simulink model "RT_TestMV"  (R2015b)
settings: Solver=FixedStepDiscrete  StartTime=0.0  StopTime=inf  FixedStep=samplePeriod  RelTol=1e-3
PreLoadFcn:
  | initialize;
  | scramInitialize;
  | KR_alpha;
  | Discrete_Compensator;
values from neighbouring files (symbols this model uses):
  a_sub = ones(DOF_sub,1)    [KR_alpha.m]
  A_sub = (dt*alpha1_sub)/(Msub-Msub*alpha3_sub)    [KR_alpha.m]
  a_sup = ones(DOF_sup,1)    [KR_alpha.m]
  A_sup = (dt*alpha1_sup)/(Msup-Msup*alpha3_sup)    [KR_alpha.m]
  a_vector = ones(DOF,1)    [KR_alpha.m]
  alpha_f_sub = rho_inf_sub/(rho_inf_sub+1)    (= 0.5)    [KR_alpha.m]
  alpha_f_sup = rho_inf_sup/(rho_inf_sup+1)    (= 0.5)    [KR_alpha.m]
  B_sub = ((1/dt)*Msub*alpha3_sub)/alpha1_sub    [KR_alpha.m]
  B_sup = ((1/dt)*Msup*alpha3_sup)/alpha1_sup    [KR_alpha.m]
  controlPeriod = 1/2048    (= 0.00048828125)    [initialize.m]
  Csub = betaKinit*Ksub    [KR_alpha.m]
  Csup = (2*0.01/w1)*Ksup    (= 0.00743030767319)    [KR_alpha.m]
  D_sub = inv(alpha1_sub)/dt    [KR_alpha.m]
  D_sup = inv(alpha1_sup)/dt    [KR_alpha.m]
  dt = samplePeriod    [KR_alpha.m]
  g = 386.089    [KR_alpha.m]
  gamma_sub = 0.5-alpha_m_sub+alpha_f_sub    (= 0.5)    [KR_alpha.m]
  gamma_sup = 0.5-alpha_m_sup+alpha_f_sup    (= 0.5)    [KR_alpha.m]
  K1 = 4.6686*K2    (= 9.3372)    [KR_alpha.m]
  K2 = 0.5*4    (= 2)    [KR_alpha.m]
  Ksub = Kstory    [KR_alpha.m]
  Msub = (0.88585/(56/450))*Mstory    (= 1.03248862309)    [KR_alpha.m]
  Msup = Mstory    (= 0.145044277356)    [KR_alpha.m]
  nAct = 4    [initialize.m]
  nDout = 4    [initialize.m]
  onesec = ceil(1/samplePeriod)    [Discrete_Compensator.m]
  samplePeriod = controlPeriod/upsampleFactor    (= 0.00048828125)    [initialize.m]
  scale_GM = 1.50    (= 1.5)    [KR_alpha.m]
  uy = 0.85    [KR_alpha.m]
undefined symbols (not defined in the file or in its folder): a, DiscIntNeverNeededParam, Gain_noise, lhpNode, stsNode
undefined symbols (not defined in the file): HybridCtrlParameters
libraries: simulink x16, slrtlib x12, xpcsystranlib x5
CloseFcn:
  | rtwprivate ssgencode ModelCloseRequest scrnet_receiver
settings Model: SimulationMode=external  ExtModeArmWhenConnect=off  Creator=mvetsch  LastModifiedBy=Analyst-UCSD
settings SolverCC: EnableConcurrentExecution=on
settings DataIOCC: LimitDataPoints=off  SaveFormat=Array  SignalLoggingSaveFormat=ModelDataLogs  SignalLoggingName=sigsOut
settings OptimizationCC: BlockReduction=off  BooleanDataType=off  OptimizeBlockIOStorage=off  BufferReuse=off  GlobalBufferReuse=off  ExpressionFolding=off  ExpressionDepthLimit=2147483647  LocalBlockOutputs=off  InitFltsAndDblsToZero=on
settings DebuggingCC: SaveWithParameterizedLinksMsg=none  UnderspecifiedInitializationDetection=Classic  MergeDetectMultiDrivingBlocksExec=none  SignalResolutionControl=TryResolveAllWithWarning  MultiTaskDSMMsg=warning  MultiTaskCondExecSysMsg=none  FcnCallInpInsideContextMsg=UseLocalSettings  StateNameClashWarn=warning
settings HardwareCC: ProdBitPerPointer=32  ProdLargestAtomicFloat=None  ProdWordSize=32  ProdLongLongMode=on  ProdHWDeviceType=Generic->32-bit x86 compatible
settings RTWCC: SystemTargetFile=slrt.tlc  TemplateMakefile=slrt_default_tmf  Description=Simulink Real-Time  RTWCompilerOptimization=on
settings SimulinkRealTimeCC: TargetFcnLib=ansi_tfl_tmw.mat  RL32LogBufSizeModifier=10000000  RL32IRQSourceModifier=Auto (PCI only)  xPCIRQSourceBoard=Scramnet_SC150+
settings ConfigComp: CovModelRefEnable=Off

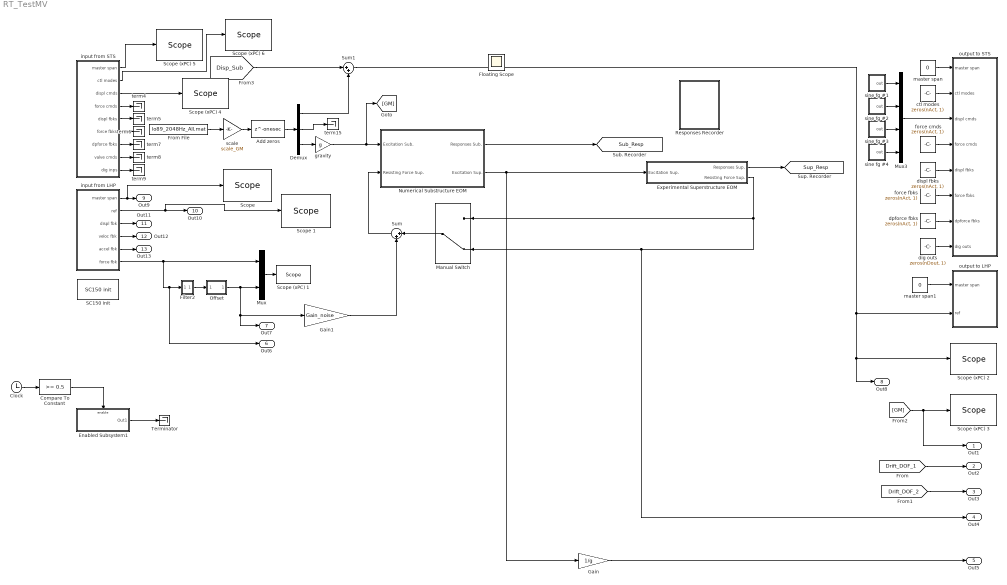
== system RT_TestMV ==
  Add zeros : Delay  DelayLength=onesec  InitialCondition=0
  Clock : Clock
  Compare To Constant : simulink/Logic and Bit Operations/Compare To Constant  relop=>=  const=0.5  OutDataTypeStr=boolean
  Demux : Demux  Outputs=3
  Enabled Subsystem1 : Subsystem  TreatAsAtomicUnit=on
  Experimental Superstructure EOM : Subsystem
  Filter2 : Subsystem
  From File : FromFile  FileName=lo89_2048Hz_All.mat  SampleTime=samplePeriod
  Gain : Gain  Gain=1/g
  Gain1 : Gain  Gain=Gain_noise
  Manual Switch : ManualSwitch  CurrentSetting=0
  Mux : Mux  Inputs=2
  Mux3 : Mux  Inputs=nAct
  Numerical Substructure EOM : Subsystem
  Offset : Subsystem  mask(Signal Offset){nS=HybridCtrlParameters.nDOF, nOffset=onesec}
      mask prompts: nS "Number of Signals: nS"; nOffset "Number of samples to initialize offset: nOffset"
      mask help:
      | Offset signal by average of signal over initial number of samples.
      | Set nOffset = -1 for no signal offset.
      mask Display: fprintf('Signal\nOffset')
  Responses Recorder : Subsystem
  SC150 init : xpcsystranlib/Shared Memory/SC150 init   node=node  pci=-1
  "Scope " : slrtlib/Displays and Logging/Scope   scopeno=8  scopetype=Target  autostart=on  viewmode=Numerical  formatstr='%15.6f'  grid=on  ylimits=[0,0]  nosamples=250  noprepostsamples=0  interleave=1  triggermode=FreeRun  triggersignal=1  trigsignalfromport=off  triggerlevel=0.0  triggerslope=Either  triggerscope=1  triggersample=0  filename=data.dat  mode=Lazy  writesize=512  autorestart=off  dynamicfilemode=off  maxwritefilesize=512*1024^2
  Scope (xPC) 1 : slrtlib/Displays and Logging/Scope   scopeno=2  scopetype=Target  autostart=on  viewmode=Graphical redraw  formatstr='%15.6f'  grid=on  ylimits=[0,0]  nosamples=1024  noprepostsamples=0  interleave=1  triggermode=FreeRun  triggersignal=1  trigsignalfromport=off  triggerlevel=0.0  triggerslope=Either  triggerscope=1  triggersample=0  filename=data.dat  mode=Lazy  writesize=512  autorestart=off  dynamicfilemode=off  maxwritefilesize=512*1024^2
  Scope (xPC) 2 : slrtlib/Displays and Logging/Scope   scopeno=3  scopetype=Target  autostart=on  viewmode=Graphical redraw  formatstr='%15.6f'  grid=on  ylimits=[0,0]  nosamples=1024  noprepostsamples=0  interleave=1  triggermode=FreeRun  triggersignal=1  trigsignalfromport=off  triggerlevel=0.0  triggerslope=Either  triggerscope=1  triggersample=0  filename=data.dat  mode=Lazy  writesize=512  autorestart=off  dynamicfilemode=off  maxwritefilesize=512*1024^2
  Scope (xPC) 3 : slrtlib/Displays and Logging/Scope   scopeno=4  scopetype=Target  autostart=on  viewmode=Graphical redraw  formatstr='%15.6f'  grid=on  ylimits=[0,0]  nosamples=1024  noprepostsamples=0  interleave=1  triggermode=FreeRun  triggersignal=1  trigsignalfromport=off  triggerlevel=0.0  triggerslope=Either  triggerscope=1  triggersample=0  filename=data.dat  mode=Lazy  writesize=512  autorestart=off  dynamicfilemode=off  maxwritefilesize=512*1024^2
  Scope (xPC) 4 : slrtlib/Displays and Logging/Scope   scopeno=1  scopetype=Target  autostart=on  viewmode=Numerical  formatstr='%15.6f'  grid=on  ylimits=[0,0]  nosamples=1024  noprepostsamples=0  interleave=1  triggermode=FreeRun  triggersignal=1  trigsignalfromport=off  triggerlevel=0.0  triggerslope=Either  triggerscope=1  triggersample=0  filename=data.dat  mode=Lazy  writesize=512  autorestart=off  dynamicfilemode=off  maxwritefilesize=512*1024^2
  Scope (xPC) 5 : slrtlib/Displays and Logging/Scope   scopeno=5  scopetype=Target  autostart=on  viewmode=Numerical  formatstr='%15.6f'  grid=on  ylimits=[0,0]  nosamples=1024  noprepostsamples=0  interleave=1  triggermode=FreeRun  triggersignal=1  trigsignalfromport=off  triggerlevel=0.0  triggerslope=Either  triggerscope=1  triggersample=0  filename=data.dat  mode=Lazy  writesize=512  autorestart=off  dynamicfilemode=off  maxwritefilesize=512*1024^2
  Scope (xPC) 6 : slrtlib/Displays and Logging/Scope   scopeno=6  scopetype=Target  autostart=on  viewmode=Numerical  formatstr='%15.6f'  grid=on  ylimits=[0,0]  nosamples=1024  noprepostsamples=0  interleave=1  triggermode=FreeRun  triggersignal=1  trigsignalfromport=off  triggerlevel=0.0  triggerslope=Either  triggerscope=1  triggersample=0  filename=data.dat  mode=Lazy  writesize=512  autorestart=off  dynamicfilemode=off  maxwritefilesize=512*1024^2
  Scope 1 : slrtlib/Displays and Logging/Scope   scopeno=7  scopetype=Target  autostart=on  viewmode=Graphical redraw  formatstr='%15.6f'  grid=on  ylimits=[0,0]  nosamples=250  noprepostsamples=0  interleave=1  triggermode=FreeRun  triggersignal=1  trigsignalfromport=off  triggerlevel=0.0  triggerslope=Either  triggerscope=1  triggersample=0  filename=data.dat  mode=Lazy  writesize=512  autorestart=off  dynamicfilemode=off  maxwritefilesize=512*1024^2
  Sum : Sum  Inputs=|++
  Sum1 : Sum  Inputs=|++
  Terminator : Terminator
  ctl modes : Constant  Value=zeros(nAct, 1)
  dig outs : Constant  Value=zeros(nDout, 1)  OutDataTypeStr=uint32
  displ fbks : Constant  Value=zeros(nAct, 1)
  dpforce fbks : Constant  Value=zeros(nAct, 1)
  force cmds : Constant  Value=zeros(nAct, 1)
  force fbks : Constant  Value=zeros(nAct, 1)
  gravity : Gain  Gain=g
  input from LHP : Subsystem
  input from STS : Subsystem
  master span : Constant  Value=0
  master span1 : Constant  Value=0
  output to LHP : Subsystem
  output to STS : Subsystem
  scale : Gain  Gain=scale_GM
  sine fg #1 : Subsystem  mask(Sine Function Generator){ampl=0.5, freq=1, spanInterval=1, samplePeriod=controlPeriod}
      mask prompts: ampl "Amplitude"; freq "Frequency (Hz)"; spanInterval "Span interval (sec)"; samplePeriod "Sample period (sec)"
  sine fg #2 : Subsystem  mask(Sine Function Generator){ampl=0.5, freq=2, spanInterval=1, samplePeriod=controlPeriod}
      mask prompts: ampl "Amplitude"; freq "Frequency (Hz)"; spanInterval "Span interval (sec)"; samplePeriod "Sample period (sec)"
  sine fg #3 : Subsystem  mask(Sine Function Generator){ampl=0.5, freq=3, spanInterval=1, samplePeriod=controlPeriod}
      mask prompts: ampl "Amplitude"; freq "Frequency (Hz)"; spanInterval "Span interval (sec)"; samplePeriod "Sample period (sec)"
  sine fg #4 : Subsystem  mask(Sine Function Generator){ampl=0.5, freq=4, spanInterval=1, samplePeriod=controlPeriod}
      mask prompts: ampl "Amplitude"; freq "Frequency (Hz)"; spanInterval "Span interval (sec)"; samplePeriod "Sample period (sec)"
  term{4..9,15} (7 alike) : Terminator
  Out1 : Outport  SampleTime=samplePeriod
  Out2 : Outport  Port=2  SampleTime=samplePeriod
  Out3 : Outport  Port=3  SampleTime=samplePeriod
  Out4 : Outport  Port=4  SampleTime=samplePeriod
  Out5 : Outport  Port=5  SampleTime=samplePeriod
  Out6 : Outport  Port=6  SampleTime=samplePeriod
  Out7 : Outport  Port=7  SampleTime=samplePeriod
  Out8 : Outport  Port=8  SampleTime=samplePeriod
  Out9 : Outport  Port=9  SampleTime=samplePeriod
  Out10 : Outport  Port=10  SampleTime=samplePeriod
  Out11 : Outport  Port=11  SampleTime=samplePeriod
  Out12 : Outport  Port=12  SampleTime=samplePeriod
  Out13 : Outport  Port=13  SampleTime=samplePeriod
  Floating Scope : Scope
  tag scope: Sub_Resp=global, Sup_Resp=global
  wires:
  master span/1 -> output to STS/1(master span)
  ctl modes/1 -> output to STS/2(ctl modes)
  force cmds/1 -> output to STS/4(force cmds)
  sine fg #1/1(out) -> Mux3/1
  sine fg #2/1(out) -> Mux3/2
  displ fbks/1 -> output to STS/5(displ fbks)
  force fbks/1 -> output to STS/6(force fbks)
  dpforce fbks/1 -> output to STS/7(dpforce fbks)
  input from STS/2(ctl modes) -> Scope (xPC) 6/1
  input from STS/4(force cmds) -> term4/1
  input from STS/5(displ fbks) -> term5/1
  input from STS/6(force fbks) -> term6/1
  input from STS/7(dpforce fbks) -> term7/1
  input from STS/8(valve cmds) -> term8/1
  input from STS/9(dig inps) -> term9/1
  dig outs/1 -> output to STS/8(dig outs)
  Mux3/1 -> output to STS/3(displ cmds)
  sine fg #3/1(out) -> Mux3/3
  sine fg #4/1(out) -> Mux3/4
  input from LHP/1(master span) -> "Scope "/1, Out9/1
  input from LHP/3(displ fbk) -> Out11/1
  input from LHP/4(veloc fbk) -> Out12/1
  input from LHP/5(accel fbk) -> Out13/1
  Mux/1 -> Scope (xPC) 1/1
  input from LHP/6(force fbk) -> Out6/1, Filter2/1(In1), Mux/1
  Numerical Substructure EOM/1(Responses Sub.) -> [Sub_Resp]
  Experimental Superstructure EOM/1(Responses Sup.) -> [Sup_Resp]
  [Drift_DOF_1] -> Out2/1
  [Drift_DOF_2] -> Out3/1
  master span1/1 -> output to LHP/1(master span)
  Filter2/1(Out1) -> Offset/1(In1)
  Offset/1(Out1) -> Out7/1, Gain1/1, Mux/2
  input from LHP/2(ref) -> Scope 1/1, Out10/1
  Experimental Superstructure EOM/2(Resisting Force Sup.) -> Manual Switch/1, Manual Switch/2, Out4/1
  From File/1 -> scale/1
  gravity/1 -> [GM], Numerical Substructure EOM/1(Excitation Sub.)
  Sum/1 -> Numerical Substructure EOM/2(Resisting Force Sup.)
  Manual Switch/1 -> Sum/1
  [GM] -> Out1/1, Scope (xPC) 3/1
  Numerical Substructure EOM/2(Excitation Sup.) -> Experimental Superstructure EOM/1(Excitation Sup.), Gain/1
  Gain1/1 -> Sum/2
  Add zeros/1 -> Demux/1
  Demux/3 -> gravity/1
  Demux/2 -> term15/1
  [Disp_Sub] -> Sum1/1
  Demux/1 -> Sum1/2
  Gain/1 -> Out5/1
  scale/1 -> Add zeros/1
  input from STS/1(master span) -> Scope (xPC) 5/1
  input from STS/3(displ cmds) -> Scope (xPC) 4/1
  Sum1/1 -> Out8/1, Scope (xPC) 2/1, output to LHP/2(ref)
  Compare To Constant/1 -> Enabled Subsystem1/Enable
  Clock/1 -> Compare To Constant/1
  Enabled Subsystem1/1(Out1) -> Terminator/1

== system RT_TestMV/Enabled Subsystem1 ==
  Enable : EnablePort
  sine fg #5 : Subsystem  mask(Sine Function Generator){ampl=1, freq=1, spanInterval=1, samplePeriod=-1}
      mask prompts: ampl "Amplitude"; freq "Frequency (Hz)"; spanInterval "Span interval (sec)"; samplePeriod "Sample period (sec)"
  Out1 : Outport
  wires:
  sine fg #5/1(out) -> Out1/1

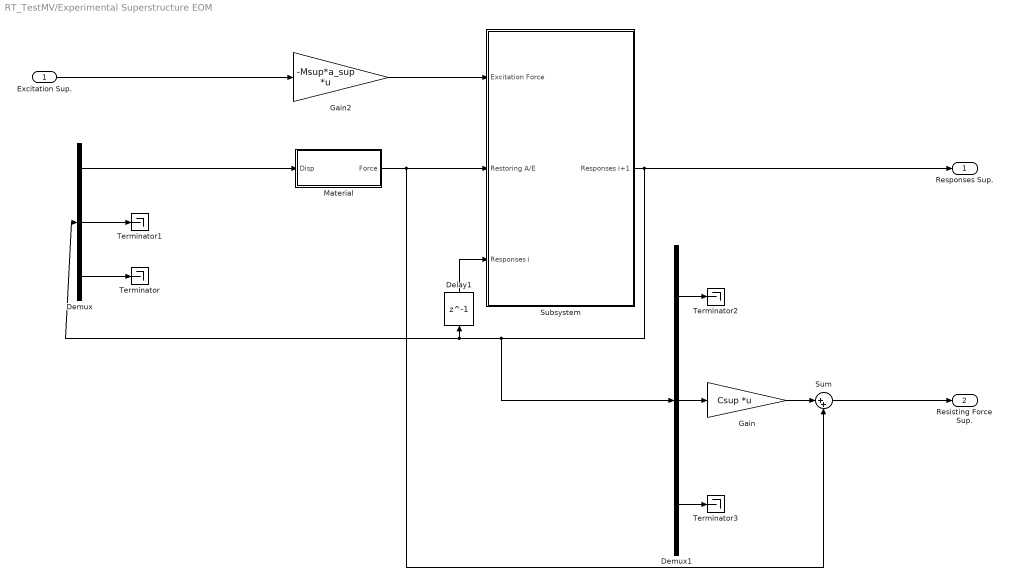
== system RT_TestMV/Experimental Superstructure EOM ==
  Excitation Sup. : Inport
  Delay1 : Delay  DelayLength=1
  Demux : Demux  Outputs=3
  Demux1 : Demux  Outputs=3
  Gain : Gain  Gain=Csup  Multiplication=Matrix(K*u) (u vector)
  Gain2 : Gain  Gain=-Msup*a_sup  Multiplication=Matrix(K*u)
  Material : Subsystem
  Subsystem : Subsystem
  Sum : Sum  Inputs=|++
  Terminator{,1..3} (4 alike) : Terminator
  Responses Sup. : Outport
  Resisting Force Sup. : Outport  Port=2
  wires:
  Subsystem/1(Responses i+1) -> Demux1/1, Demux/1, Delay1/1, Responses Sup./1
  Excitation Sup./1 -> Gain2/1
  Demux1/2 -> Gain/1
  Sum/1 -> Resisting Force Sup./1
  Demux/1 -> Material/1(Disp)
  Demux/3 -> Terminator/1
  Demux/2 -> Terminator1/1
  Demux1/1 -> Terminator2/1
  Demux1/3 -> Terminator3/1
  Gain/1 -> Sum/1
  Delay1/1 -> Subsystem/3(Responses i)
  Material/1(Force) -> Sum/2, Subsystem/2(Restoring A/E)
  Gain2/1 -> Subsystem/1(Excitation Force)

== system RT_TestMV/Filter2 ==
  In1 : Inport
  MovingAverage Filter2 : DiscreteFir  Coefficients=1/numSample*ones(1,numSample)  mask(Moving Average Filter){numSample=7}
      mask prompts: numSample "Number of Samples: numSample"
      mask help:
      | Moving average filter by using discrete FIR filter.
      | Set numSample = 1 for no filtering.
      mask Display: fprintf('MovingAverage\nFilter')
  Out1 : Outport
  wires:
  In1/1 -> MovingAverage Filter2/1
  MovingAverage Filter2/1 -> Out1/1

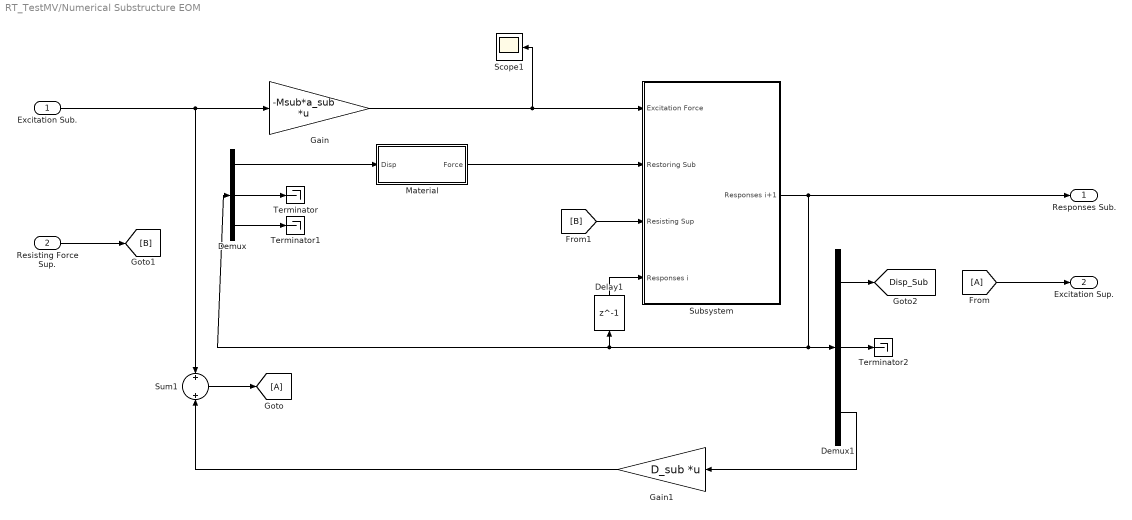
== system RT_TestMV/Numerical Substructure EOM ==
  Excitation Sub. : Inport
  Resisting Force Sup. : Inport  Port=2
  Delay1 : Delay  DelayLength=1
  Demux : Demux  Outputs=3
  Demux1 : Demux  Outputs=3
  Gain : Gain  Gain=-Msub*a_sub  Multiplication=Matrix(K*u)
  Gain1 : Gain  Gain=D_sub  Multiplication=Matrix(K*u) (u vector)
  Material : Subsystem
  Scope1 : Scope
  Subsystem : Subsystem
  Sum1 : Sum  Inputs=+||+
  Terminator : Terminator
  Terminator1 : Terminator
  Terminator2 : Terminator
  Responses Sub. : Outport
  Excitation Sup. : Outport  Port=2
  tag scope: Disp_Sub=global
  wires:
  Gain/1 -> Scope1/1, Subsystem/1(Excitation Force)
  Subsystem/1(Responses i+1) -> Demux/1, Delay1/1, Demux1/1, Responses Sub./1
  Demux/1 -> Material/1(Disp)
  Excitation Sub./1 -> Sum1/1, Gain/1
  Demux1/3 -> Gain1/1
  Demux/2 -> Terminator/1
  Demux/3 -> Terminator1/1
  Demux1/1 -> [Disp_Sub]
  Delay1/1 -> Subsystem/4(Responses i)
  Material/1(Force) -> Subsystem/2(Restoring Sub)
  Gain1/1 -> Sum1/2
  Demux1/2 -> Terminator2/1
  Sum1/1 -> [A]
  [A] -> Excitation Sup./1
  Resisting Force Sup./1 -> [B]
  [B] -> Subsystem/3(Resisting Sup)

== system RT_TestMV/Offset ==
  In1 : Inport
  Constant : Constant  Value=zeros(1,nS)
  Counter : simulink/Sources/Counter Free-Running  NumBits=32  tsamp=-1
  Data Store Memory : DataStoreMemory  DataStoreName=x0  InitialValue=zeros(1,nS)  OutDataTypeStr=double
  Data Store Read : DataStoreRead  DataStoreName=x0  SampleTime=controlPeriod
  If : If  IfExpression=u1 < nOffset  ShowElse=off
  If Action : Subsystem  TreatAsAtomicUnit=on
  Sum1 : Sum  Inputs=+-|  SaturateOnIntegerOverflow=on  InputSameDT=on  OutDataTypeStr=Inherit: Same as first input
  Switch : Switch  Threshold=nOffset  SaturateOnIntegerOverflow=on  InputSameDT=on
  typeConv2 : DataTypeConversion  OutDataTypeStr=double  SaturateOnIntegerOverflow=on  RndMeth=Zero
  Out1 : Outport
  wires:
  Switch/1 -> Out1/1
  Sum1/1 -> Switch/1
  Data Store Read/1 -> Sum1/2
  In1/1 -> If Action/1(In1), Sum1/1
  Constant/1 -> Switch/3
  Counter/1 -> typeConv2/1
  If/1 -> If Action/Action
  typeConv2/1 -> Switch/2, If/1

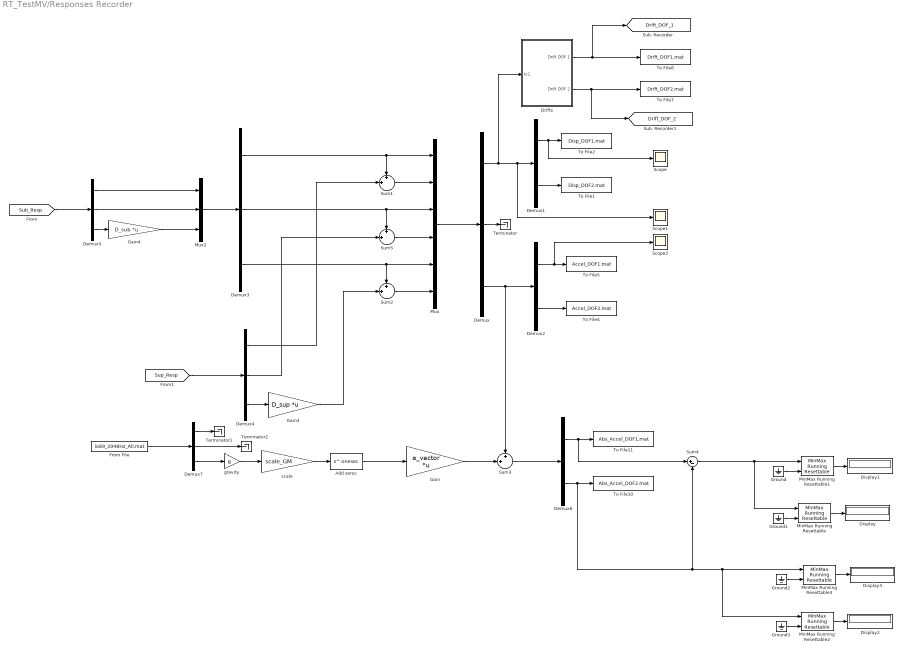
== system RT_TestMV/Responses Recorder ==
  Add zeros : Delay  DelayLength=onesec  InitialCondition=0
  Demux{,3..5,7} (5 alike) : Demux  Outputs=3
  Demux1 : Demux  Outputs=2
  Demux2 : Demux  Outputs=2
  Demux6 : Demux  Outputs=2
  Display{,1..3} (4 alike) : Display
  Drifts : Subsystem
  From File : FromFile  FileName=lo89_2048Hz_All.mat  SampleTime=samplePeriod
  Gain : Gain  Gain=a_vector  Multiplication=Matrix(K*u)
  Gain3 : Gain  Gain=D_sup  Multiplication=Matrix(K*u) (u vector)
  Gain4 : Gain  Gain=D_sub  Multiplication=Matrix(K*u) (u vector)
  Ground{,1..3} (4 alike) : Ground
  MinMax Running Resettable : simulink/Math Operations/MinMax Running Resettable  Function=max  vinit=0.0
  MinMax Running Resettable1 : simulink/Math Operations/MinMax Running Resettable  Function=min  vinit=0.0
  MinMax Running Resettable2 : simulink/Math Operations/MinMax Running Resettable  Function=max  vinit=0.0
  MinMax Running Resettable3 : simulink/Math Operations/MinMax Running Resettable  Function=min  vinit=0.0
  Mux : Mux  Inputs=6
  Mux2 : Mux  Inputs=3
  Scope : Scope
  Scope1 : Scope
  Scope2 : Scope
  Sum{1..3,5} (4 alike) : Sum  Inputs=+|+||
  Sum4 : Sum  Inputs=|+-
  Terminator : Terminator
  Terminator1 : Terminator
  Terminator2 : Terminator
  To File1 : ToFile  Filename=Disp_DOF2.mat
  To File10 : ToFile  Filename=Abs_Accel_DOF2.mat
  To File11 : ToFile  Filename=Abs_Accel_DOF1.mat
  To File2 : ToFile  Filename=Disp_DOF1.mat
  To File4 : ToFile  Filename=Accel_DOF2.mat
  To File5 : ToFile  Filename=Accel_DOF1.mat
  To File7 : ToFile  Filename=Drift_DOF2.mat  MatrixName=Drift_DOF2
  To File8 : ToFile  Filename=Drift_DOF1.mat  MatrixName=Drift_DOF1
  gravity : Gain  Gain=g
  scale : Gain  Gain=scale_GM
  tag scope: Drift_DOF_1=global, Drift_DOF_2=global
  wires:
  Demux1/2 -> To File1/1
  Demux2/1 -> Scope2/1, To File5/1
  Demux/3 -> Sum3/1, Demux2/1
  Demux1/1 -> Scope/1, To File2/1
  Demux/1 -> Drifts/1(In1), Scope1/1, Demux1/1
  [Sup_Resp] -> Demux4/1
  Mux/1 -> Demux/1
  Demux3/3 -> Sum2/1, Mux/5
  Demux4/3 -> Gain3/1
  Sum2/1 -> Mux/6
  Gain3/1 -> Sum2/2
  [Sub_Resp] -> Demux5/1
  Demux5/2 -> Mux2/2
  Demux5/1 -> Mux2/1
  Demux5/3 -> Gain4/1
  Gain4/1 -> Mux2/3
  Mux2/1 -> Demux3/1
  Demux/2 -> Terminator/1
  MinMax Running Resettable/1 -> Display/1
  MinMax Running Resettable1/1 -> Display1/1
  Ground/1 -> MinMax Running Resettable1/2
  Ground1/1 -> MinMax Running Resettable/2
  Demux2/2 -> To File4/1
  MinMax Running Resettable2/1 -> Display2/1
  MinMax Running Resettable3/1 -> Display3/1
  Ground2/1 -> MinMax Running Resettable3/2
  Ground3/1 -> MinMax Running Resettable2/2
  Drifts/1(Drift DOF 1) -> [Drift_DOF_1], To File8/1
  Drifts/2(Drift DOF 2) -> [Drift_DOF_2], To File7/1
  gravity/1 -> scale/1
  Gain/1 -> Sum3/2
  Sum3/1 -> Demux6/1
  scale/1 -> Add zeros/1
  Demux3/1 -> Sum1/1, Mux/1
  Demux4/1 -> Sum1/2
  Sum1/1 -> Mux/2
  Demux3/2 -> Sum5/1, Mux/3
  Demux4/2 -> Sum5/2
  Sum5/1 -> Mux/4
  Demux6/1 -> Sum4/1, To File11/1
  Demux6/2 -> Sum4/2, MinMax Running Resettable2/1, MinMax Running Resettable3/1, To File10/1
  Sum4/1 -> MinMax Running Resettable/1, MinMax Running Resettable1/1
  Add zeros/1 -> Gain/1
  Demux7/3 -> gravity/1
  From File/1 -> Demux7/1
  Demux7/1 -> Terminator1/1
  Demux7/2 -> Terminator2/1

== system RT_TestMV/input from LHP ==
  SC150 read : xpcsystranlib/Shared Memory/SC150 read   partition=lhpNode.Partitions(3:end)  errorport=off  ts=controlPeriod  pci=-1
  SC150 unpack : slrtlib/Shared Memory/Shared Memory Unpack   partition=lhpNode.Partitions(3:end)
  typeConv{1..6} (6 alike) : DataTypeConversion  OutDataTypeStr=double  SaturateOnIntegerOverflow=on  RndMeth=Zero
  master span : Outport
  ref : Outport  Port=2
  displ fbk : Outport  Port=3
  veloc fbk : Outport  Port=4
  accel fbk : Outport  Port=5
  force fbk : Outport  Port=6
  wires:
  SC150 unpack/6 -> typeConv6/1
  SC150 unpack/5 -> typeConv5/1
  SC150 unpack/4 -> typeConv4/1
  SC150 unpack/3 -> typeConv3/1
  SC150 unpack/2 -> typeConv2/1
  typeConv6/1 -> force fbk/1
  typeConv5/1 -> accel fbk/1
  typeConv4/1 -> veloc fbk/1
  typeConv3/1 -> displ fbk/1
  typeConv1/1 -> master span/1
  SC150 read/1 -> SC150 unpack/1
  typeConv2/1 -> ref/1
  SC150 unpack/1 -> typeConv1/1

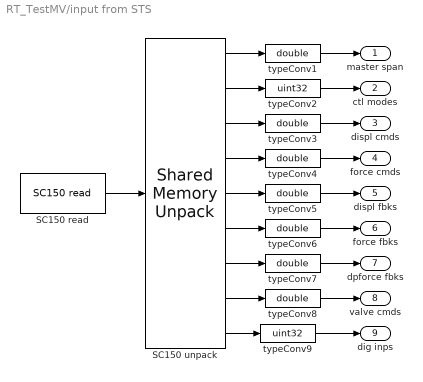
== system RT_TestMV/input from STS ==
  SC150 read : xpcsystranlib/Shared Memory/SC150 read   partition=stsNode.Partitions(9:end)  errorport=off  ts=controlPeriod  pci=-1
  SC150 unpack : slrtlib/Shared Memory/Shared Memory Unpack   partition=stsNode.Partitions(9:end)
  typeConv{1,3..8} (7 alike) : DataTypeConversion  OutDataTypeStr=double  SaturateOnIntegerOverflow=on  RndMeth=Zero
  typeConv2 : DataTypeConversion  OutDataTypeStr=uint32  SaturateOnIntegerOverflow=on  RndMeth=Zero
  typeConv9 : DataTypeConversion  OutDataTypeStr=uint32  SaturateOnIntegerOverflow=on  RndMeth=Zero
  master span : Outport
  ctl modes : Outport  Port=2
  displ cmds : Outport  Port=3
  force cmds : Outport  Port=4
  displ fbks : Outport  Port=5
  force fbks : Outport  Port=6
  dpforce fbks : Outport  Port=7
  valve cmds : Outport  Port=8
  dig inps : Outport  Port=9
  wires:
  SC150 unpack/8 -> typeConv8/1
  SC150 unpack/7 -> typeConv7/1
  SC150 unpack/6 -> typeConv6/1
  SC150 unpack/5 -> typeConv5/1
  SC150 unpack/4 -> typeConv4/1
  SC150 unpack/2 -> typeConv2/1
  typeConv2/1 -> ctl modes/1
  SC150 read/1 -> SC150 unpack/1
  typeConv1/1 -> master span/1
  typeConv3/1 -> displ cmds/1
  typeConv4/1 -> force cmds/1
  typeConv5/1 -> displ fbks/1
  typeConv6/1 -> force fbks/1
  typeConv7/1 -> dpforce fbks/1
  typeConv8/1 -> valve cmds/1
  SC150 unpack/9 -> typeConv9/1
  typeConv9/1 -> dig inps/1
  SC150 unpack/3 -> typeConv3/1
  SC150 unpack/1 -> typeConv1/1

== system RT_TestMV/output to LHP ==
  master span : Inport
  ref : Inport  Port=2
  SC150 pack : slrtlib/Shared Memory/Shared Memory Pack   partition=lhpNode.Partitions(1:2)
  SC150 write : xpcsystranlib/Shared Memory/SC150 write   partition=lhpNode.Partitions(1:2)  errorport=off  ts=controlPeriod  pci=-1
  typeConv1 : DataTypeConversion  OutDataTypeStr=single  SaturateOnIntegerOverflow=on  RndMeth=Zero
  typeConv2 : DataTypeConversion  OutDataTypeStr=single  SaturateOnIntegerOverflow=on  RndMeth=Zero
  wires:
  master span/1 -> typeConv1/1
  SC150 pack/1 -> SC150 write/1
  ref/1 -> typeConv2/1
  typeConv1/1 -> SC150 pack/1
  typeConv2/1 -> SC150 pack/2

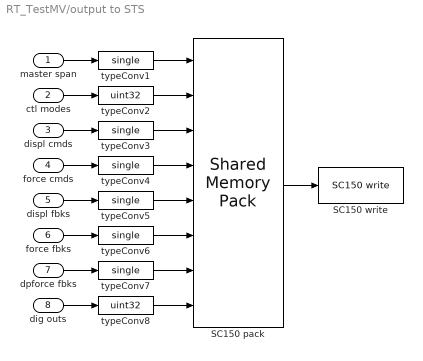
== system RT_TestMV/output to STS ==
  master span : Inport
  ctl modes : Inport  Port=2
  displ cmds : Inport  Port=3
  force cmds : Inport  Port=4
  displ fbks : Inport  Port=5
  force fbks : Inport  Port=6
  dpforce fbks : Inport  Port=7
  dig outs : Inport  Port=8
  SC150 pack : slrtlib/Shared Memory/Shared Memory Pack   partition=stsNode.Partitions(1:8)
  SC150 write : xpcsystranlib/Shared Memory/SC150 write   partition=stsNode.Partitions(1:8)  errorport=off  ts=controlPeriod  pci=-1
  typeConv{1,3..7} (6 alike) : DataTypeConversion  OutDataTypeStr=single  SaturateOnIntegerOverflow=on  RndMeth=Zero
  typeConv2 : DataTypeConversion  OutDataTypeStr=uint32  SaturateOnIntegerOverflow=on  RndMeth=Zero
  typeConv8 : DataTypeConversion  OutDataTypeStr=uint32  SaturateOnIntegerOverflow=on  RndMeth=Zero
  wires:
  typeConv4/1 -> SC150 pack/4
  typeConv3/1 -> SC150 pack/3
  typeConv2/1 -> SC150 pack/2
  typeConv1/1 -> SC150 pack/1
  ctl modes/1 -> typeConv2/1
  displ cmds/1 -> typeConv3/1
  SC150 pack/1 -> SC150 write/1
  master span/1 -> typeConv1/1
  force cmds/1 -> typeConv4/1
  displ fbks/1 -> typeConv5/1
  force fbks/1 -> typeConv6/1
  dpforce fbks/1 -> typeConv7/1
  typeConv5/1 -> SC150 pack/5
  typeConv6/1 -> SC150 pack/6
  typeConv7/1 -> SC150 pack/7
  typeConv8/1 -> SC150 pack/8
  dig outs/1 -> typeConv8/1

== system RT_TestMV/sine fg #1 ==
  Product : Product  SaturateOnIntegerOverflow=on  InputSameDT=on  OutDataTypeStr=Inherit: Same as first input
  integrator : DiscreteIntegrator  SampleTime=-1  LimitOutput=on  UpperSaturationLimit=1  LowerSaturationLimit=0  ICPrevOutput=DiscIntNeverNeededParam  ICPrevScaledInput=DiscIntNeverNeededParam
  sine : Sin  Amplitude=ampl  Frequency=2 * pi * freq  SampleTime=samplePeriod
  span rate : Constant  Value=1/spanInterval
  out : Outport
  wires:
  Product/1 -> out/1
  sine/1 -> Product/1
  span rate/1 -> integrator/1
  integrator/1 -> Product/2

== system RT_TestMV/sine fg #2 ==
  Product : Product  SaturateOnIntegerOverflow=on  InputSameDT=on  OutDataTypeStr=Inherit: Same as first input
  integrator : DiscreteIntegrator  SampleTime=-1  LimitOutput=on  UpperSaturationLimit=1  LowerSaturationLimit=0  ICPrevOutput=DiscIntNeverNeededParam  ICPrevScaledInput=DiscIntNeverNeededParam
  sine : Sin  Amplitude=ampl  Frequency=2 * pi * freq  SampleTime=samplePeriod
  span rate : Constant  Value=1/spanInterval
  out : Outport
  wires:
  integrator/1 -> Product/2
  span rate/1 -> integrator/1
  sine/1 -> Product/1
  Product/1 -> out/1

== system RT_TestMV/sine fg #3 ==
  Product : Product  SaturateOnIntegerOverflow=on  InputSameDT=on  OutDataTypeStr=Inherit: Same as first input
  integrator : DiscreteIntegrator  SampleTime=-1  LimitOutput=on  UpperSaturationLimit=1  LowerSaturationLimit=0  ICPrevOutput=DiscIntNeverNeededParam  ICPrevScaledInput=DiscIntNeverNeededParam
  sine : Sin  Amplitude=ampl  Frequency=2 * pi * freq  SampleTime=samplePeriod
  span rate : Constant  Value=1/spanInterval
  out : Outport
  wires:
  Product/1 -> out/1
  sine/1 -> Product/1
  span rate/1 -> integrator/1
  integrator/1 -> Product/2

== system RT_TestMV/sine fg #4 ==
  Product : Product  SaturateOnIntegerOverflow=on  InputSameDT=on  OutDataTypeStr=Inherit: Same as first input
  integrator : DiscreteIntegrator  SampleTime=-1  LimitOutput=on  UpperSaturationLimit=1  LowerSaturationLimit=0  ICPrevOutput=DiscIntNeverNeededParam  ICPrevScaledInput=DiscIntNeverNeededParam
  sine : Sin  Amplitude=ampl  Frequency=2 * pi * freq  SampleTime=samplePeriod
  span rate : Constant  Value=1/spanInterval
  out : Outport
  wires:
  integrator/1 -> Product/2
  span rate/1 -> integrator/1
  sine/1 -> Product/1
  Product/1 -> out/1

== system RT_TestMV/Enabled Subsystem1/sine fg #5 ==
  Product : Product  SaturateOnIntegerOverflow=on  InputSameDT=on  OutDataTypeStr=Inherit: Same as first input
  integrator : DiscreteIntegrator  SampleTime=-1  LimitOutput=on  UpperSaturationLimit=1  LowerSaturationLimit=0  ICPrevOutput=DiscIntNeverNeededParam  ICPrevScaledInput=DiscIntNeverNeededParam
  sine : Sin  Amplitude=ampl  Frequency=2 * pi * freq  SampleTime=samplePeriod
  span rate : Constant  Value=1/spanInterval
  out : Outport
  wires:
  integrator/1 -> Product/2
  span rate/1 -> integrator/1
  sine/1 -> Product/1
  Product/1 -> out/1

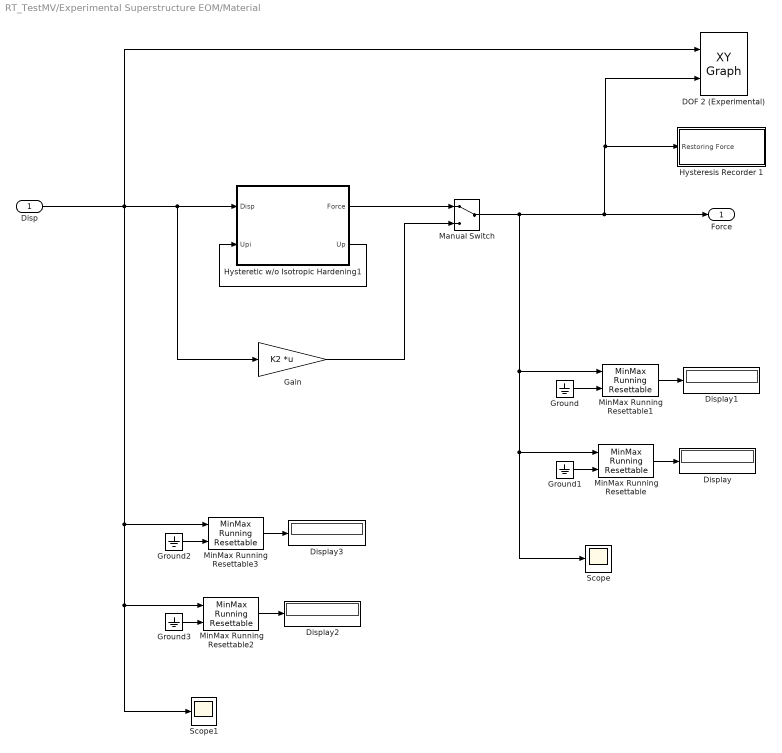
== system RT_TestMV/Experimental Superstructure EOM/Material ==
  Disp : Inport
  DOF 2 (Experimental) : simulink/Sinks/XY Graph  xmin=-6  xmax=6  ymin=-25  ymax=25  st=-1
  Display{,1..3} (4 alike) : Display
  Gain : Gain  Gain=K2  Multiplication=Matrix(K*u) (u vector)
  Ground{,1..3} (4 alike) : Ground
  Hysteresis Recorder 1 : Subsystem
  Hysteretic w/o Isotropic Hardening1 : Subsystem
  Manual Switch : ManualSwitch
  MinMax Running Resettable : simulink/Math Operations/MinMax Running Resettable  Function=max  vinit=0.0
  MinMax Running Resettable1 : simulink/Math Operations/MinMax Running Resettable  Function=min  vinit=0.0
  MinMax Running Resettable2 : simulink/Math Operations/MinMax Running Resettable  Function=max  vinit=0.0
  MinMax Running Resettable3 : simulink/Math Operations/MinMax Running Resettable  Function=min  vinit=0.0
  Scope : Scope
  Scope1 : Scope
  Force : Outport
  wires:
  Hysteretic w/o Isotropic Hardening1/2(Up) -> Hysteretic w/o Isotropic Hardening1/2(Upi)
  Hysteretic w/o Isotropic Hardening1/1(Force) -> Manual Switch/1
  Gain/1 -> Manual Switch/2
  MinMax Running Resettable2/1 -> Display2/1
  Ground/1 -> MinMax Running Resettable1/2
  Ground2/1 -> MinMax Running Resettable3/2
  Ground1/1 -> MinMax Running Resettable/2
  MinMax Running Resettable1/1 -> Display1/1
  MinMax Running Resettable/1 -> Display/1
  Ground3/1 -> MinMax Running Resettable2/2
  Manual Switch/1 -> MinMax Running Resettable1/1, MinMax Running Resettable/1, Scope/1, DOF 2 (Experimental)/2, Hysteresis Recorder 1/1(Restoring Force), Force/1
  MinMax Running Resettable3/1 -> Display3/1
  Disp/1 -> DOF 2 (Experimental)/1, MinMax Running Resettable3/1, MinMax Running Resettable2/1, Scope1/1, Gain/1, Hysteretic w/o Isotropic Hardening1/1(Disp)

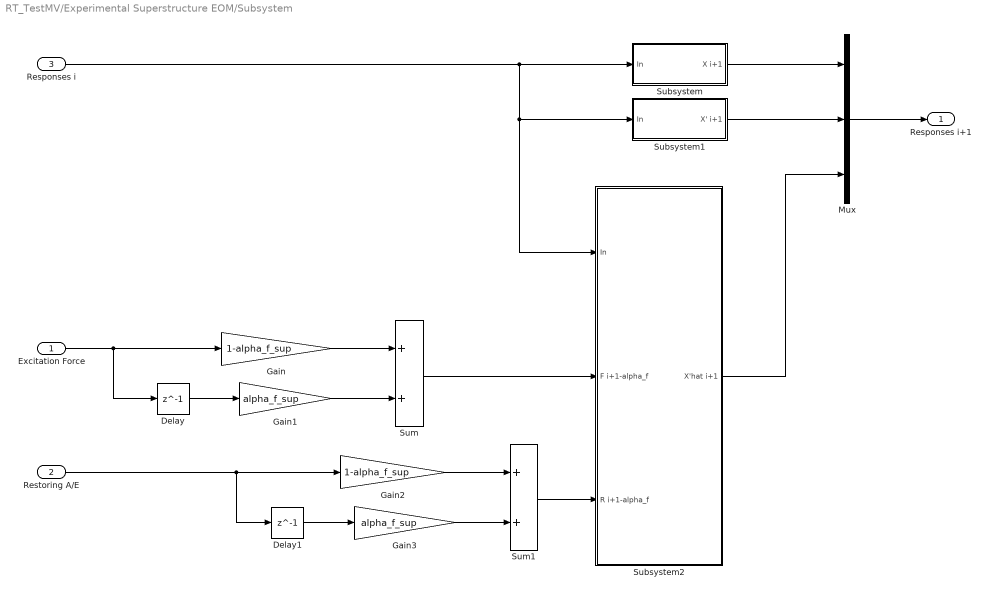
== system RT_TestMV/Experimental Superstructure EOM/Subsystem ==
  Excitation Force : Inport
  Restoring A/E : Inport  Port=2
  Responses i : Inport  Port=3
  Delay : Delay  DelayLength=1
  Delay1 : Delay  DelayLength=1
  Gain : Gain  Gain=1-alpha_f_sup
  Gain1 : Gain  Gain=alpha_f_sup
  Gain2 : Gain  Gain=1-alpha_f_sup
  Gain3 : Gain  Gain=alpha_f_sup
  Mux : Mux  Inputs=3
  Subsystem : Subsystem
  Subsystem1 : Subsystem
  Subsystem2 : Subsystem
  Sum : Sum
  Sum1 : Sum
  Responses i+1 : Outport
  wires:
  Excitation Force/1 -> Delay/1, Gain/1
  Delay/1 -> Gain1/1
  Gain/1 -> Sum/1
  Gain1/1 -> Sum/2
  Sum/1 -> Subsystem2/2(F i+1-alpha_f)
  Mux/1 -> Responses i+1/1
  Subsystem1/1(X' i+1) -> Mux/2
  Subsystem/1(X i+1) -> Mux/1
  Subsystem2/1(X'hat i+1) -> Mux/3
  Delay1/1 -> Gain3/1
  Gain2/1 -> Sum1/1
  Gain3/1 -> Sum1/2
  Sum1/1 -> Subsystem2/3(R i+1-alpha_f)
  Responses i/1 -> Subsystem2/1(In), Subsystem1/1(In), Subsystem/1(In)
  Restoring A/E/1 -> Delay1/1, Gain2/1

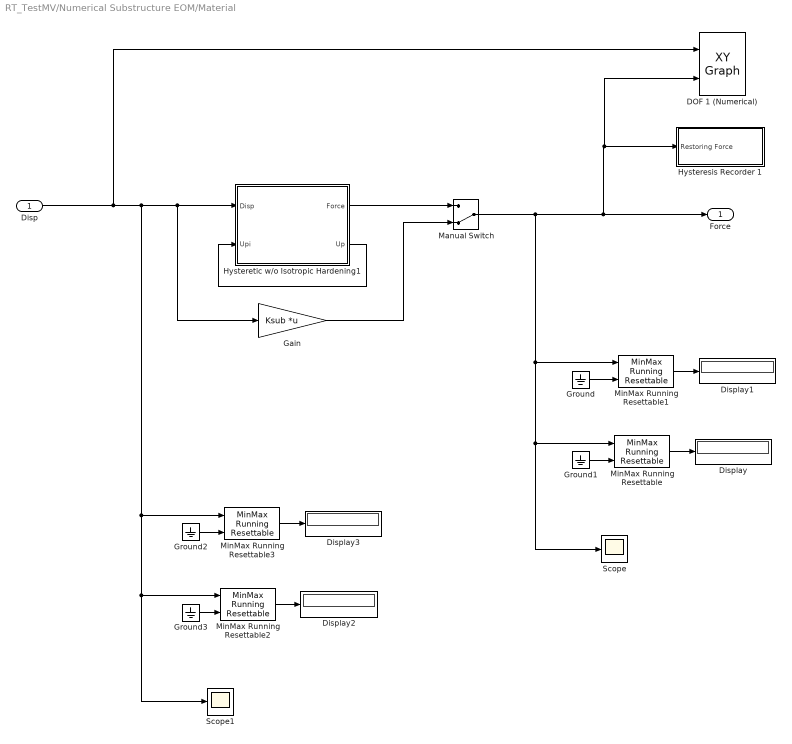
== system RT_TestMV/Numerical Substructure EOM/Material ==
  Disp : Inport
  DOF 1 (Numerical) : simulink/Sinks/XY Graph  xmin=-1  xmax=1  ymin=-35  ymax=35  st=-1
  Display{,1..3} (4 alike) : Display
  Gain : Gain  Gain=Ksub  Multiplication=Matrix(K*u) (u vector)
  Ground{,1..3} (4 alike) : Ground
  Hysteresis Recorder 1 : Subsystem
  Hysteretic w/o Isotropic Hardening1 : Subsystem
  Manual Switch : ManualSwitch  CurrentSetting=0
  MinMax Running Resettable : simulink/Math Operations/MinMax Running Resettable  Function=max  vinit=0.0
  MinMax Running Resettable1 : simulink/Math Operations/MinMax Running Resettable  Function=min  vinit=0.0
  MinMax Running Resettable2 : simulink/Math Operations/MinMax Running Resettable  Function=max  vinit=0.0
  MinMax Running Resettable3 : simulink/Math Operations/MinMax Running Resettable  Function=min  vinit=0.0
  Scope : Scope
  Scope1 : Scope
  Force : Outport
  wires:
  Hysteretic w/o Isotropic Hardening1/2(Up) -> Hysteretic w/o Isotropic Hardening1/2(Upi)
  Hysteretic w/o Isotropic Hardening1/1(Force) -> Manual Switch/1
  Gain/1 -> Manual Switch/2
  Ground2/1 -> MinMax Running Resettable3/2
  Ground/1 -> MinMax Running Resettable1/2
  MinMax Running Resettable2/1 -> Display2/1
  Manual Switch/1 -> MinMax Running Resettable1/1, MinMax Running Resettable/1, Scope/1, DOF 1 (Numerical)/2, Hysteresis Recorder 1/1(Restoring Force), Force/1
  MinMax Running Resettable3/1 -> Display3/1
  MinMax Running Resettable1/1 -> Display1/1
  Ground1/1 -> MinMax Running Resettable/2
  Disp/1 -> MinMax Running Resettable3/1, MinMax Running Resettable2/1, Scope1/1, Gain/1, Hysteretic w/o Isotropic Hardening1/1(Disp), DOF 1 (Numerical)/1
  Ground3/1 -> MinMax Running Resettable2/2
  MinMax Running Resettable/1 -> Display/1

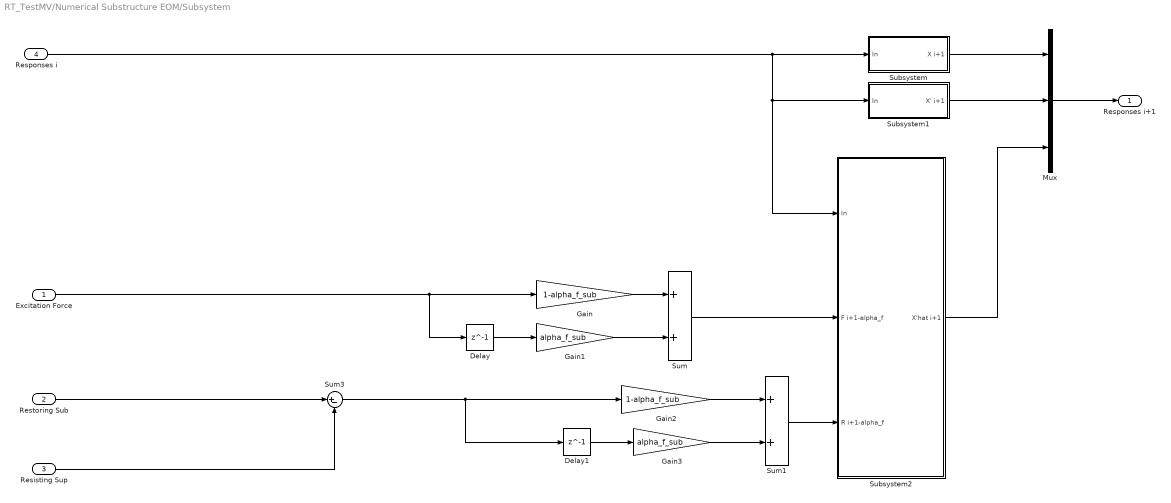
== system RT_TestMV/Numerical Substructure EOM/Subsystem ==
  Excitation Force : Inport
  Restoring Sub : Inport  Port=2
  Resisting Sup : Inport  Port=3
  Responses i : Inport  Port=4
  Delay : Delay  DelayLength=1
  Delay1 : Delay  DelayLength=1
  Gain : Gain  Gain=1-alpha_f_sub
  Gain1 : Gain  Gain=alpha_f_sub
  Gain2 : Gain  Gain=1-alpha_f_sub
  Gain3 : Gain  Gain=alpha_f_sub
  Mux : Mux  Inputs=3
  Subsystem : Subsystem
  Subsystem1 : Subsystem
  Subsystem2 : Subsystem
  Sum : Sum
  Sum1 : Sum
  Sum3 : Sum  Inputs=|+-
  Responses i+1 : Outport
  wires:
  Excitation Force/1 -> Delay/1, Gain/1
  Delay/1 -> Gain1/1
  Gain/1 -> Sum/1
  Gain1/1 -> Sum/2
  Sum/1 -> Subsystem2/2(F i+1-alpha_f)
  Mux/1 -> Responses i+1/1
  Subsystem1/1(X' i+1) -> Mux/2
  Subsystem/1(X i+1) -> Mux/1
  Subsystem2/1(X'hat i+1) -> Mux/3
  Delay1/1 -> Gain3/1
  Gain2/1 -> Sum1/1
  Gain3/1 -> Sum1/2
  Sum1/1 -> Subsystem2/3(R i+1-alpha_f)
  Responses i/1 -> Subsystem2/1(In), Subsystem1/1(In), Subsystem/1(In)
  Sum3/1 -> Delay1/1, Gain2/1
  Restoring Sub/1 -> Sum3/1
  Resisting Sup/1 -> Sum3/2

== system RT_TestMV/Offset/If Action ==
  In1 : Inport
  Action Port : ActionPort  PropagateVarSize=During execution  ActionType=then
  Data Store Read : DataStoreRead  DataStoreName=x0  SampleTime=controlPeriod
  Data Store Write : DataStoreWrite  DataStoreName=x0
  Gain : Gain  Gain=1/nOffset  SaturateOnIntegerOverflow=on  OutDataTypeStr=Inherit: Same as input  ParamDataTypeStr=Inherit: Same as input
  Sum : Sum  Inputs=|++  SaturateOnIntegerOverflow=on  InputSameDT=on  OutDataTypeStr=Inherit: Same as first input
  wires:
  Data Store Read/1 -> Sum/2
  Sum/1 -> Data Store Write/1
  Gain/1 -> Sum/1
  In1/1 -> Gain/1

== system RT_TestMV/Responses Recorder/Drifts ==
  In1 : Inport
  Demux : Demux  Outputs=2
  Sum5 : Sum  Inputs=-|+||
  Drift DOF 1 : Outport
  Drift DOF 2 : Outport  Port=2
  wires:
  In1/1 -> Demux/1
  Demux/2 -> Sum5/2
  Demux/1 -> Sum5/1, Drift DOF 1/1
  Sum5/1 -> Drift DOF 2/1

== system RT_TestMV/Experimental Superstructure EOM/Material/Hysteresis Recorder 1 ==
  Restoring Force : Inport
  To File2 : ToFile  Filename=Restoring_DOF2.mat  MatrixName=Restoring_DOF2
  wires:
  Restoring Force/1 -> To File2/1

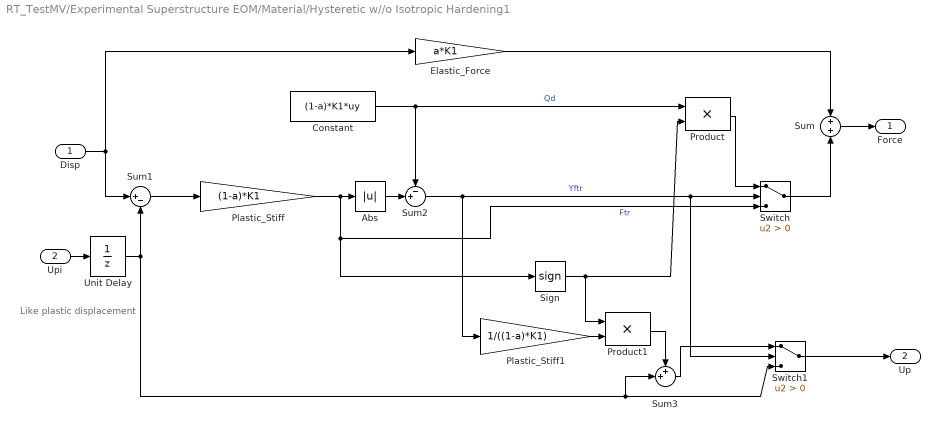
== system RT_TestMV/Experimental Superstructure EOM/Material/Hysteretic w//o Isotropic Hardening1 ==
  note: Like plastic displacement
  Disp : Inport
  Upi : Inport  Port=2
  Abs : Abs  SaturateOnIntegerOverflow=on
  Constant : Constant  Value=(1-a)*K1*uy
  Elastic_Force : Gain  Gain=a*K1  SaturateOnIntegerOverflow=on  OutDataTypeStr=Inherit: Same as input  ParamDataTypeStr=Inherit: Same as input
  Plastic_Stiff : Gain  Gain=(1-a)*K1  SaturateOnIntegerOverflow=on  OutDataTypeStr=Inherit: Same as input  ParamDataTypeStr=Inherit: Same as input
  Plastic_Stiff1 : Gain  Gain=1/((1-a)*K1)  SaturateOnIntegerOverflow=on  OutDataTypeStr=Inherit: Same as input  ParamDataTypeStr=Inherit: Same as input
  Product : Product  SaturateOnIntegerOverflow=on  OutDataTypeStr=Inherit: Same as first input
  Product1 : Product  SaturateOnIntegerOverflow=on  OutDataTypeStr=Inherit: Same as first input
  Sign : Signum
  Sum : Sum  Inputs=+|+  SaturateOnIntegerOverflow=on  InputSameDT=on  OutDataTypeStr=Inherit: Same as first input
  Sum1 : Sum  Inputs=|+-  SaturateOnIntegerOverflow=on
  Sum2 : Sum  Inputs=-+|  SaturateOnIntegerOverflow=on
  Sum3 : Sum  Inputs=++|  SaturateOnIntegerOverflow=on
  Switch : Switch  Criteria=u2 > Threshold  SaturateOnIntegerOverflow=on
  Switch1 : Switch  Criteria=u2 > Threshold  SaturateOnIntegerOverflow=on
  Unit Delay : UnitDelay  SampleTime=-1
  Force : Outport
  Up : Outport  Port=2
  wires:
  Elastic_Force/1 -> Sum/1
  Disp/1 -> Sum1/1, Elastic_Force/1
  Sum/1 -> Force/1
  Upi/1 -> Unit Delay/1
  Sum1/1 -> Plastic_Stiff/1
  Plastic_Stiff/1 -> Abs/1, Switch/3, Sign/1  "Ftr"
  Constant/1 -> Sum2/1, Product/1  "Qd"
  Sum2/1 -> Switch/2, Switch1/2, Plastic_Stiff1/1  "Yftr"
  Product/1 -> Switch/1
  Switch/1 -> Sum/2
  Switch1/1 -> Up/1
  Sum3/1 -> Switch1/1
  Product1/1 -> Sum3/1
  Plastic_Stiff1/1 -> Product1/2
  Unit Delay/1 -> Sum1/2, Sum3/2, Switch1/3
  Sign/1 -> Product1/1, Product/2
  Abs/1 -> Sum2/2

== system RT_TestMV/Experimental Superstructure EOM/Subsystem/Subsystem ==
  In : Inport
  Demux : Demux  Outputs=3
  Gain : Gain  Gain=dt
  Gain1 : Gain  Gain=(0.5+gamma_sup)*dt
  Sum1 : Sum  Inputs=+++
  X i+1 : Outport
  wires:
  In/1 -> Demux/1
  Demux/3 -> Gain1/1
  Demux/2 -> Gain/1
  Demux/1 -> Sum1/1
  Gain/1 -> Sum1/2
  Gain1/1 -> Sum1/3
  Sum1/1 -> X i+1/1

== system RT_TestMV/Experimental Superstructure EOM/Subsystem/Subsystem1 ==
  In : Inport
  Demux : Demux  Outputs=3
  Sum : Sum  Inputs=|++
  Terminator : Terminator
  X' i+1 : Outport
  wires:
  In/1 -> Demux/1
  Sum/1 -> X' i+1/1
  Demux/3 -> Sum/2
  Demux/2 -> Sum/1
  Demux/1 -> Terminator/1

== system RT_TestMV/Experimental Superstructure EOM/Subsystem/Subsystem2 ==
  In : Inport
  F i+1-alpha_f : Inport  Port=2
  R i+1-alpha_f : Inport  Port=3
  Demux : Demux  Outputs=3
  Gain : Gain  Gain=B_sup  Multiplication=Matrix(K*u) (u vector)
  Gain1 : Gain  Gain=1-alpha_f_sup
  Gain2 : Gain  Gain=Csup  Multiplication=Matrix(K*u) (u vector)
  Gain3 : Gain  Gain=A_sup  Multiplication=Matrix(K*u) (u vector)
  Sum : Sum  Inputs=+---
  Sum1 : Sum  Inputs=|++
  Terminator : Terminator
  X'hat i+1 : Outport
  wires:
  In/1 -> Demux/1
  Demux/3 -> Gain/1, Gain1/1
  Gain/1 -> Sum/4
  Demux/2 -> Sum1/1
  Sum1/1 -> Gain2/1
  Gain1/1 -> Sum1/2
  Gain2/1 -> Sum/2
  F i+1-alpha_f/1 -> Sum/1
  R i+1-alpha_f/1 -> Sum/3
  Sum/1 -> Gain3/1
  Gain3/1 -> X'hat i+1/1
  Demux/1 -> Terminator/1

== system RT_TestMV/Numerical Substructure EOM/Material/Hysteresis Recorder 1 ==
  Restoring Force : Inport
  To File2 : ToFile  Filename=Restoring_DOF1.mat  MatrixName=Restoring_DOF1
  wires:
  Restoring Force/1 -> To File2/1

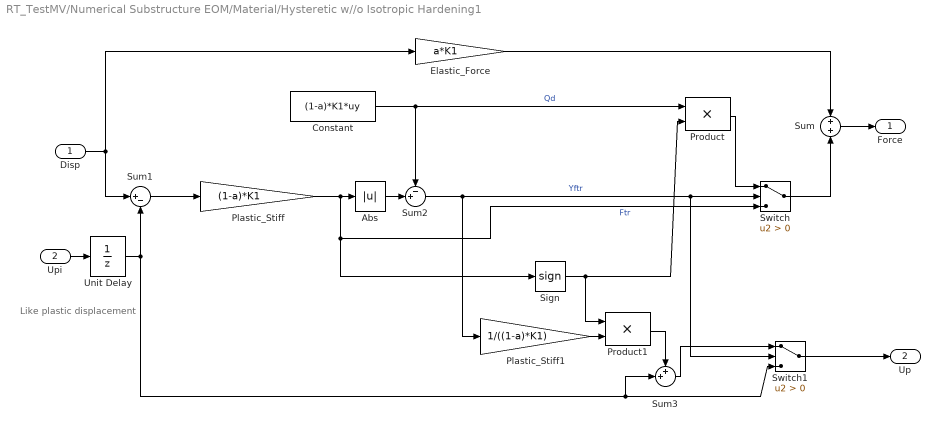
== system RT_TestMV/Numerical Substructure EOM/Material/Hysteretic w//o Isotropic Hardening1 ==
  note: Like plastic displacement
  Disp : Inport
  Upi : Inport  Port=2
  Abs : Abs  SaturateOnIntegerOverflow=on
  Constant : Constant  Value=(1-a)*K1*uy
  Elastic_Force : Gain  Gain=a*K1  SaturateOnIntegerOverflow=on  OutDataTypeStr=Inherit: Same as input  ParamDataTypeStr=Inherit: Same as input
  Plastic_Stiff : Gain  Gain=(1-a)*K1  SaturateOnIntegerOverflow=on  OutDataTypeStr=Inherit: Same as input  ParamDataTypeStr=Inherit: Same as input
  Plastic_Stiff1 : Gain  Gain=1/((1-a)*K1)  SaturateOnIntegerOverflow=on  OutDataTypeStr=Inherit: Same as input  ParamDataTypeStr=Inherit: Same as input
  Product : Product  SaturateOnIntegerOverflow=on  OutDataTypeStr=Inherit: Same as first input
  Product1 : Product  SaturateOnIntegerOverflow=on  OutDataTypeStr=Inherit: Same as first input
  Sign : Signum
  Sum : Sum  Inputs=+|+  SaturateOnIntegerOverflow=on  InputSameDT=on  OutDataTypeStr=Inherit: Same as first input
  Sum1 : Sum  Inputs=|+-  SaturateOnIntegerOverflow=on
  Sum2 : Sum  Inputs=-+|  SaturateOnIntegerOverflow=on
  Sum3 : Sum  Inputs=++|  SaturateOnIntegerOverflow=on
  Switch : Switch  Criteria=u2 > Threshold  SaturateOnIntegerOverflow=on
  Switch1 : Switch  Criteria=u2 > Threshold  SaturateOnIntegerOverflow=on
  Unit Delay : UnitDelay  SampleTime=-1
  Force : Outport
  Up : Outport  Port=2
  wires:
  Elastic_Force/1 -> Sum/1
  Disp/1 -> Sum1/1, Elastic_Force/1
  Sum/1 -> Force/1
  Upi/1 -> Unit Delay/1
  Sum1/1 -> Plastic_Stiff/1
  Plastic_Stiff/1 -> Abs/1, Switch/3, Sign/1  "Ftr"
  Constant/1 -> Sum2/1, Product/1  "Qd"
  Sum2/1 -> Switch/2, Switch1/2, Plastic_Stiff1/1  "Yftr"
  Product/1 -> Switch/1
  Switch/1 -> Sum/2
  Switch1/1 -> Up/1
  Sum3/1 -> Switch1/1
  Product1/1 -> Sum3/1
  Plastic_Stiff1/1 -> Product1/2
  Unit Delay/1 -> Sum1/2, Sum3/2, Switch1/3
  Sign/1 -> Product1/1, Product/2
  Abs/1 -> Sum2/2

== system RT_TestMV/Numerical Substructure EOM/Subsystem/Subsystem ==
  In : Inport
  Demux : Demux  Outputs=3
  Gain : Gain  Gain=dt
  Gain1 : Gain  Gain=(0.5+gamma_sub)*dt
  Sum1 : Sum  Inputs=+++
  X i+1 : Outport
  wires:
  In/1 -> Demux/1
  Demux/3 -> Gain1/1
  Demux/2 -> Gain/1
  Demux/1 -> Sum1/1
  Gain/1 -> Sum1/2
  Gain1/1 -> Sum1/3
  Sum1/1 -> X i+1/1

== system RT_TestMV/Numerical Substructure EOM/Subsystem/Subsystem1 ==
  In : Inport
  Demux : Demux  Outputs=3
  Sum : Sum  Inputs=|++
  Terminator : Terminator
  X' i+1 : Outport
  wires:
  In/1 -> Demux/1
  Sum/1 -> X' i+1/1
  Demux/3 -> Sum/2
  Demux/2 -> Sum/1
  Demux/1 -> Terminator/1

== system RT_TestMV/Numerical Substructure EOM/Subsystem/Subsystem2 ==
  In : Inport
  F i+1-alpha_f : Inport  Port=2
  R i+1-alpha_f : Inport  Port=3
  Demux : Demux  Outputs=3
  Gain : Gain  Gain=B_sub  Multiplication=Matrix(K*u) (u vector)
  Gain1 : Gain  Gain=1-alpha_f_sub
  Gain2 : Gain  Gain=Csub  Multiplication=Matrix(K*u) (u vector)
  Gain3 : Gain  Gain=A_sub  Multiplication=Matrix(K*u) (u vector)
  Sum : Sum  Inputs=+---
  Sum1 : Sum  Inputs=|++
  Terminator : Terminator
  X'hat i+1 : Outport
  wires:
  In/1 -> Demux/1
  Demux/3 -> Gain/1, Gain1/1
  Gain/1 -> Sum/4
  Demux/2 -> Sum1/1
  Sum1/1 -> Gain2/1
  Gain1/1 -> Sum1/2
  Gain2/1 -> Sum/2
  F i+1-alpha_f/1 -> Sum/1
  R i+1-alpha_f/1 -> Sum/3
  Sum/1 -> Gain3/1
  Gain3/1 -> X'hat i+1/1
  Demux/1 -> Terminator/1
